simulink model "SPGF_FSK_0000_R2019b"  (R2019b)
settings: Solver=ode3  SolverName=ode4  StartTime=0.0  StopTime=1.4  FixedStep=50e-6/50  RelTol=1e-3  EnableMultiTasking=on
undefined symbols (not defined in the file): D11, Delta
libraries: powerlib x2544, powerlib_meascontrol x204, simulink x24
(part 8 of 33)

== system SPGF_FSK_0000_R2019b/K8/fault ==
  Add : Sum  Inputs=+-
  Arcing : Subsystem  TreatAsAtomicUnit=on
  Constant2 : Constant  Value=FaultPhase
  Control : Product  Inputs=***
  Count Limiter : Subsystem
  Demux : Demux  Outputs=2
  Fault Interruption : Subsystem
  Fault A : Constant  Value=FaultA
  Fault A1 : Constant  Value=0
  Fault A2 : Constant  Value=LimitArcNum
  Fault A3 : Constant  Value=AddTimeDelay
  Fault B : Constant  Value=FaultB
  Fault C : Constant  Value=FaultC
  Ground1 : powerlib/Elements/Ground  LConnTagsString=a
  Ideal Switch A : powerlib/Power Electronics/Ideal Switch  Ron=FaultResistance  Lon=0  IC=0  Rs=SnubberResistance  Cs=SnubberCapacitance  Measurements=on
  Ideal Switch B : powerlib/Power Electronics/Ideal Switch  Ron=FaultResistance  Lon=0  IC=0  Rs=SnubberResistance  Cs=SnubberCapacitance  Measurements=on
  Ideal Switch C : powerlib/Power Electronics/Ideal Switch  Ron=FaultResistance  Lon=0  IC=0  Rs=SnubberResistance  Cs=SnubberCapacitance  Measurements=on
  Mux : Mux  Inputs=2
  Product : Product
  Product1 : Product
  Product2 : Product
  Rground : powerlib/Elements/Series RLC Branch  LConnTagsString=__new0  RConnTagsString=__new0  BranchType=R  Resistance=GroundResistance  Inductance=0  SetiL0=off  InitialCurrent=0  Capacitance=inf  Setx0=off  InitialVoltage=0  Measurements=None
  SW : MultiPortSwitch  DataPortForDefault=Additional data port
  SW_Limit : Switch  Criteria=u2 > Threshold  Threshold=0.5
  SW_TD : Switch  Criteria=u2 > Threshold  Threshold=0.5
  Step : Step  Time=EndFaultTime  SampleTime=0
  Step1 : Step  Time=BeginFaultTime  SampleTime=0
  Time Delay : Subsystem
  A : PMIOPort  Side=Left
  B : PMIOPort  Port=2  Side=Left
  C : PMIOPort  Port=3  Side=Left
  wires:
  Demux/1 -> [I]
  Control/1 -> Time Delay/2(Control), SW_TD/3
  Count Limiter/2(O) -> SW_Limit/1
  Fault A2/1 -> SW_Limit/2
  Arcing/1(O) -> Control/2
  Mux/1 -> Arcing/1(I)
  [V] -> Mux/2
  [I] -> Mux/1
  Add/1 -> Control/1, Arcing/Enable
  Step/1 -> Add/2
  Step1/1 -> Add/1
  Product2/1 -> Ideal Switch C/1
  Fault C/1 -> Product2/2
  Product1/1 -> Ideal Switch B/1
  Fault B/1 -> Product1/2
  Product/1 -> Ideal Switch A/1
  Fault A/1 -> Product/2
  Ideal Switch C/1 -> SW/4
  Ideal Switch B/1 -> SW/3
  Ideal Switch A/1 -> SW/2
  Fault A1/1 -> SW/5
  SW/1 -> Demux/1
  Constant2/1 -> SW/1
  Fault Interruption/1(O) -> Control/3
  SW_Limit/1 -> Product/1, Product1/1, Product2/1
  Fault A3/1 -> SW_TD/2
  SW_TD/1 -> SW_Limit/3, Count Limiter/1(I)
  Count Limiter/1(Count) -> Time Delay/1(Count)
  Time Delay/1(O) -> SW_TD/1
  Demux/2 -> [V]
  connections:
  Ground1/LConn1 -- Rground/RConn1
  Ideal Switch B/RConn1 -- Ideal Switch A/RConn1 -- Rground/LConn1 -- Ideal Switch C/RConn1
  Ideal Switch B/LConn1 -- B/RConn1
  Ideal Switch A/LConn1 -- A/RConn1
  Ideal Switch C/LConn1 -- C/RConn1

== system SPGF_FSK_0000_R2019b/K8/meas ==
  Add : Sum  Inputs=+++
  GainI : Gain
  GainI0 : Gain
  I A: : powerlib/Measurements/Current Measurement  PhasorSimulation=off  OutputType=Complex  PSBequivalent=0
  I B: : powerlib/Measurements/Current Measurement  PhasorSimulation=off  OutputType=Complex  PSBequivalent=0
  I C: : powerlib/Measurements/Current Measurement  PhasorSimulation=off  OutputType=Complex  PSBequivalent=0
  Mux : Mux  Inputs=3
  A : PMIOPort  Side=Left
  B : PMIOPort  Port=2  Side=Left
  C : PMIOPort  Port=3  Side=Left
  a : PMIOPort  Port=4  Side=Right
  b : PMIOPort  Port=5  Side=Right
  c : PMIOPort  Port=6  Side=Right
  tag scope: CT3I0_K8=global, CTIabc_K8=global
  wires:
  I A:/1 -> Mux/1, Add/1
  I B:/1 -> Mux/2, Add/2
  I C:/1 -> Mux/3, Add/3
  Add/1 -> GainI0/1
  GainI0/1 -> [CT3I0_K8]
  Mux/1 -> GainI/1
  GainI/1 -> [CTIabc_K8]
  connections:
  I C:/RConn1 -- c/RConn1
  I B:/RConn1 -- b/RConn1
  a/RConn1 -- I A:/RConn1
  I A:/LConn1 -- A/RConn1
  I C:/LConn1 -- C/RConn1
  I B:/LConn1 -- B/RConn1

== system SPGF_FSK_0000_R2019b/K9/fault ==
  Add : Sum  Inputs=+-
  Arcing : Subsystem  TreatAsAtomicUnit=on
  Constant2 : Constant  Value=FaultPhase
  Control : Product  Inputs=***
  Count Limiter : Subsystem
  Demux : Demux  Outputs=2
  Fault Interruption : Subsystem
  Fault A : Constant  Value=FaultA
  Fault A1 : Constant  Value=0
  Fault A2 : Constant  Value=LimitArcNum
  Fault A3 : Constant  Value=AddTimeDelay
  Fault B : Constant  Value=FaultB
  Fault C : Constant  Value=FaultC
  Ground1 : powerlib/Elements/Ground  LConnTagsString=a
  Ideal Switch A : powerlib/Power Electronics/Ideal Switch  Ron=FaultResistance  Lon=0  IC=0  Rs=SnubberResistance  Cs=SnubberCapacitance  Measurements=on
  Ideal Switch B : powerlib/Power Electronics/Ideal Switch  Ron=FaultResistance  Lon=0  IC=0  Rs=SnubberResistance  Cs=SnubberCapacitance  Measurements=on
  Ideal Switch C : powerlib/Power Electronics/Ideal Switch  Ron=FaultResistance  Lon=0  IC=0  Rs=SnubberResistance  Cs=SnubberCapacitance  Measurements=on
  Mux : Mux  Inputs=2
  Product : Product
  Product1 : Product
  Product2 : Product
  Rground : powerlib/Elements/Series RLC Branch  LConnTagsString=__new0  RConnTagsString=__new0  BranchType=R  Resistance=GroundResistance  Inductance=0  SetiL0=off  InitialCurrent=0  Capacitance=inf  Setx0=off  InitialVoltage=0  Measurements=None
  SW : MultiPortSwitch  DataPortForDefault=Additional data port
  SW_Limit : Switch  Criteria=u2 > Threshold  Threshold=0.5
  SW_TD : Switch  Criteria=u2 > Threshold  Threshold=0.5
  Step : Step  Time=EndFaultTime  SampleTime=0
  Step1 : Step  Time=BeginFaultTime  SampleTime=0
  Time Delay : Subsystem
  A : PMIOPort  Side=Left
  B : PMIOPort  Port=2  Side=Left
  C : PMIOPort  Port=3  Side=Left
  wires:
  Demux/2 -> [V]
  Time Delay/1(O) -> SW_TD/1
  Count Limiter/1(Count) -> Time Delay/1(Count)
  SW_TD/1 -> Count Limiter/1(I), SW_Limit/3
  Fault A3/1 -> SW_TD/2
  SW_Limit/1 -> Product2/1, Product1/1, Product/1
  Fault Interruption/1(O) -> Control/3
  Constant2/1 -> SW/1
  SW/1 -> Demux/1
  Fault A1/1 -> SW/5
  Ideal Switch A/1 -> SW/2
  Ideal Switch B/1 -> SW/3
  Ideal Switch C/1 -> SW/4
  Fault A/1 -> Product/2
  Product/1 -> Ideal Switch A/1
  Fault B/1 -> Product1/2
  Product1/1 -> Ideal Switch B/1
  Fault C/1 -> Product2/2
  Product2/1 -> Ideal Switch C/1
  Step1/1 -> Add/1
  Step/1 -> Add/2
  Add/1 -> Arcing/Enable, Control/1
  [I] -> Mux/1
  [V] -> Mux/2
  Mux/1 -> Arcing/1(I)
  Arcing/1(O) -> Control/2
  Fault A2/1 -> SW_Limit/2
  Count Limiter/2(O) -> SW_Limit/1
  Control/1 -> SW_TD/3, Time Delay/2(Control)
  Demux/1 -> [I]
  connections:
  Ideal Switch C/LConn1 -- C/RConn1
  Ideal Switch A/LConn1 -- A/RConn1
  Ideal Switch B/LConn1 -- B/RConn1
  Ideal Switch C/RConn1 -- Rground/LConn1 -- Ideal Switch A/RConn1 -- Ideal Switch B/RConn1
  Ground1/LConn1 -- Rground/RConn1

== system SPGF_FSK_0000_R2019b/K9/meas ==
  Add : Sum  Inputs=+++
  GainI : Gain
  GainI0 : Gain
  I A: : powerlib/Measurements/Current Measurement  PhasorSimulation=off  OutputType=Complex  PSBequivalent=0
  I B: : powerlib/Measurements/Current Measurement  PhasorSimulation=off  OutputType=Complex  PSBequivalent=0
  I C: : powerlib/Measurements/Current Measurement  PhasorSimulation=off  OutputType=Complex  PSBequivalent=0
  Mux : Mux  Inputs=3
  A : PMIOPort  Side=Left
  B : PMIOPort  Port=2  Side=Left
  C : PMIOPort  Port=3  Side=Left
  a : PMIOPort  Port=4  Side=Right
  b : PMIOPort  Port=5  Side=Right
  c : PMIOPort  Port=6  Side=Right
  tag scope: CT3I0_K9=global, CTIabc_K9=global
  wires:
  GainI/1 -> [CTIabc_K9]
  Mux/1 -> GainI/1
  GainI0/1 -> [CT3I0_K9]
  Add/1 -> GainI0/1
  I C:/1 -> Add/3, Mux/3
  I B:/1 -> Add/2, Mux/2
  I A:/1 -> Add/1, Mux/1
  connections:
  I B:/LConn1 -- B/RConn1
  I C:/LConn1 -- C/RConn1
  I A:/LConn1 -- A/RConn1
  a/RConn1 -- I A:/RConn1
  I B:/RConn1 -- b/RConn1
  I C:/RConn1 -- c/RConn1

== system SPGF_FSK_0000_R2019b/TP11/Nonlinear Load ==
  Cap : powerlib/Elements/Series RLC Branch  LConnTagsString=__new0  RConnTagsString=__new0  BranchType=C  Resistance=34  Inductance=1.04  SetiL0=off  InitialCurrent=0  Capacitance=4e-06  Setx0=off  InitialVoltage=0  Measurements=None
  Cap1 : powerlib/Elements/Series RLC Branch  LConnTagsString=__new0  RConnTagsString=__new0  BranchType=C  Resistance=34  Inductance=1.04  SetiL0=off  InitialCurrent=0  Capacitance=4e-06  Setx0=off  InitialVoltage=0  Measurements=None
  Cap2 : powerlib/Elements/Series RLC Branch  LConnTagsString=__new0  RConnTagsString=__new0  BranchType=C  Resistance=34  Inductance=1.04  SetiL0=off  InitialCurrent=0  Capacitance=4e-06  Setx0=off  InitialVoltage=0  Measurements=None
  Ground : powerlib/Elements/Ground  LConnTagsString=a
  RL : powerlib/Elements/Series RLC Branch  LConnTagsString=__new0  RConnTagsString=__new0  BranchType=RL  Resistance=58  Inductance=1.04  SetiL0=off  InitialCurrent=0  Capacitance=1e-6  Setx0=off  InitialVoltage=0  Measurements=None
  RL1 : powerlib/Elements/Series RLC Branch  LConnTagsString=__new0  RConnTagsString=__new0  BranchType=RL  Resistance=40  Inductance=1.04  SetiL0=off  InitialCurrent=0  Capacitance=1e-6  Setx0=off  InitialVoltage=0  Measurements=None
  RL2 : powerlib/Elements/Series RLC Branch  LConnTagsString=__new0  RConnTagsString=__new0  BranchType=RL  Resistance=40  Inductance=1.04  SetiL0=off  InitialCurrent=0  Capacitance=1e-6  Setx0=off  InitialVoltage=0  Measurements=None
  Universal Bridge : powerlib/Power Electronics/Universal Bridge  Arms=2  SnubberResistance=1e5  SnubberCapacitance=inf  Device=Diodes  Ron=1e-3  Lon=0  ForwardVoltages="[  0  0  ]"  ForwardVoltage=-160  GTOparameters=[ 10e-6 , 20e-6 ]  IGBTparameters=[ 1e-6 , 2e-6 ]  Measurements=None  Measurements_2=None  converterType=Rectifier
  Universal Bridge1 : powerlib/Power Electronics/Universal Bridge  Arms=2  SnubberResistance=1e5  SnubberCapacitance=inf  Device=Diodes  Ron=1e-3  Lon=0  ForwardVoltages="[  0  0  ]"  ForwardVoltage=-160  GTOparameters=[ 10e-6 , 20e-6 ]  IGBTparameters=[ 1e-6 , 2e-6 ]  Measurements=None  Measurements_2=None  converterType=Rectifier
  Universal Bridge2 : powerlib/Power Electronics/Universal Bridge  Arms=2  SnubberResistance=1e5  SnubberCapacitance=inf  Device=Diodes  Ron=1e-3  Lon=0  ForwardVoltages="[  0  0  ]"  ForwardVoltage=-160  GTOparameters=[ 10e-6 , 20e-6 ]  IGBTparameters=[ 1e-6 , 2e-6 ]  Measurements=None  Measurements_2=None  converterType=Rectifier
  A : PMIOPort  Side=Left
  B : PMIOPort  Port=2  Side=Left
  C : PMIOPort  Port=3  Side=Left
  connections:
  Cap/LConn1 -- Universal Bridge/RConn1 -- RL/LConn1
  Cap/RConn1 -- RL/RConn1 -- Universal Bridge/RConn2
  Cap1/LConn1 -- Universal Bridge1/RConn1 -- RL1/LConn1
  Universal Bridge1/RConn2 -- RL1/RConn1 -- Cap1/RConn1
  Cap2/LConn1 -- Universal Bridge2/RConn1 -- RL2/LConn1
  Cap2/RConn1 -- Universal Bridge2/RConn2 -- RL2/RConn1
  Universal Bridge/LConn1 -- A/RConn1
  Universal Bridge1/LConn1 -- B/RConn1
  Universal Bridge2/LConn1 -- C/RConn1
  Ground/LConn1 -- Universal Bridge/LConn2 -- Universal Bridge1/LConn2 -- Universal Bridge2/LConn2

== system SPGF_FSK_0000_R2019b/TP11/Nonlinear Load 3ph ==
  Cap : powerlib/Elements/Series RLC Branch  LConnTagsString=__new0  RConnTagsString=__new0  BranchType=C  Resistance=34  Inductance=1.04  SetiL0=off  InitialCurrent=0  Capacitance=4e-06  Setx0=off  InitialVoltage=0  Measurements=None
  RL : powerlib/Elements/Series RLC Branch  LConnTagsString=__new0  RConnTagsString=__new0  BranchType=RL  Resistance=58  Inductance=1.04  SetiL0=off  InitialCurrent=0  Capacitance=1e-6  Setx0=off  InitialVoltage=0  Measurements=None
  Universal Bridge : powerlib/Power Electronics/Universal Bridge  Arms=3  SnubberResistance=1e5  SnubberCapacitance=inf  Device=Diodes  Ron=1e-3  Lon=0  ForwardVoltages="[  0  0  ]"  ForwardVoltage=-160  GTOparameters=[ 10e-6 , 20e-6 ]  IGBTparameters=[ 1e-6 , 2e-6 ]  Measurements=None  Measurements_2=None  converterType=Rectifier
  A : PMIOPort  Side=Left
  B : PMIOPort  Port=2  Side=Left
  C : PMIOPort  Port=3  Side=Left
  connections:
  Universal Bridge/RConn1 -- RL/LConn1 -- Cap/LConn1
  Cap/RConn1 -- Universal Bridge/RConn2 -- RL/RConn1
  Universal Bridge/LConn2 -- B/RConn1
  C/RConn1 -- Universal Bridge/LConn3
  A/RConn1 -- Universal Bridge/LConn1

== system SPGF_FSK_0000_R2019b/TP11/Q ==
  breaker : Subsystem  Commented=on  mask{SwitchA=off, SwitchB=off, SwitchC=off, InitialStatus=[1 1 1], BreakerResistance=0.0001, SnubberResistance=1e6, SnubberCapacitance=inf, TransitionTimes=[0.5 0.7], ShiftTimes=[0 0 0]}
      mask prompts: SwitchA "Switching of phase A"; SwitchB "Switching of phase B"; SwitchC "Switching of phase C"; InitialStatus "Initial status of phase breaker [A, B, C]"; BreakerResistance "Breaker resistance Ron (ohms) :"; SnubberResistance "Snubbers resistance Rp (ohms) :"; SnubberCapacitance "Snubbers capacitance Cp (F) :"; TransitionTimes "Transition times (s) :"; ShiftTimes "Time differences for switch [tA, tB, tC] (s) :"
      mask init: same as SPGF_FSK_0000_R2019b/Feed/Q/breaker
      mask Display:
      | % port_label('input',1,'Iabc');
      | 
      | port_label('lconn',1,'A');
      | port_label('lconn',2,'B');
      | port_label('lconn',3,'C');
      | 
      | port_label('rconn',1,'a');
      | port_label('rconn',2,'b');
      | port_label('rconn',3,'c');
      | 
      | disp('   Q    ');
  meas : Subsystem
  shunt : Subsystem
  A : PMIOPort  Side=Right
  B : PMIOPort  Port=2  Side=Right
  C : PMIOPort  Port=3  Side=Right
  a : PMIOPort  Port=4  Side=Left
  b : PMIOPort  Port=5  Side=Left
  c : PMIOPort  Port=6  Side=Left
  connections:
  shunt/LConn3 -- C/RConn1 -- breaker/LConn3
  shunt/LConn2 -- B/RConn1 -- breaker/LConn2
  A/RConn1 -- shunt/LConn1 -- breaker/LConn1
  meas/RConn1 -- a/RConn1
  meas/RConn2 -- b/RConn1
  meas/RConn3 -- c/RConn1
  meas/LConn3 -- breaker/RConn3 -- shunt/RConn3
  meas/LConn2 -- breaker/RConn2 -- shunt/RConn2
  meas/LConn1 -- breaker/RConn1 -- shunt/RConn1

== system SPGF_FSK_0000_R2019b/TP12/Nonlinear Load ==
  Cap : powerlib/Elements/Series RLC Branch  LConnTagsString=__new0  RConnTagsString=__new0  BranchType=C  Resistance=34  Inductance=1.04  SetiL0=off  InitialCurrent=0  Capacitance=4e-06  Setx0=off  InitialVoltage=0  Measurements=None
  Cap1 : powerlib/Elements/Series RLC Branch  LConnTagsString=__new0  RConnTagsString=__new0  BranchType=C  Resistance=34  Inductance=1.04  SetiL0=off  InitialCurrent=0  Capacitance=4e-06  Setx0=off  InitialVoltage=0  Measurements=None
  Cap2 : powerlib/Elements/Series RLC Branch  LConnTagsString=__new0  RConnTagsString=__new0  BranchType=C  Resistance=34  Inductance=1.04  SetiL0=off  InitialCurrent=0  Capacitance=4e-06  Setx0=off  InitialVoltage=0  Measurements=None
  Ground : powerlib/Elements/Ground  LConnTagsString=a
  RL : powerlib/Elements/Series RLC Branch  LConnTagsString=__new0  RConnTagsString=__new0  BranchType=RL  Resistance=58  Inductance=1.04  SetiL0=off  InitialCurrent=0  Capacitance=1e-6  Setx0=off  InitialVoltage=0  Measurements=None
  RL1 : powerlib/Elements/Series RLC Branch  LConnTagsString=__new0  RConnTagsString=__new0  BranchType=RL  Resistance=40  Inductance=1.04  SetiL0=off  InitialCurrent=0  Capacitance=1e-6  Setx0=off  InitialVoltage=0  Measurements=None
  RL2 : powerlib/Elements/Series RLC Branch  LConnTagsString=__new0  RConnTagsString=__new0  BranchType=RL  Resistance=40  Inductance=1.04  SetiL0=off  InitialCurrent=0  Capacitance=1e-6  Setx0=off  InitialVoltage=0  Measurements=None
  Universal Bridge : powerlib/Power Electronics/Universal Bridge  Arms=2  SnubberResistance=1e5  SnubberCapacitance=inf  Device=Diodes  Ron=1e-3  Lon=0  ForwardVoltages="[  0  0  ]"  ForwardVoltage=-160  GTOparameters=[ 10e-6 , 20e-6 ]  IGBTparameters=[ 1e-6 , 2e-6 ]  Measurements=None  Measurements_2=None  converterType=Rectifier
  Universal Bridge1 : powerlib/Power Electronics/Universal Bridge  Arms=2  SnubberResistance=1e5  SnubberCapacitance=inf  Device=Diodes  Ron=1e-3  Lon=0  ForwardVoltages="[  0  0  ]"  ForwardVoltage=-160  GTOparameters=[ 10e-6 , 20e-6 ]  IGBTparameters=[ 1e-6 , 2e-6 ]  Measurements=None  Measurements_2=None  converterType=Rectifier
  Universal Bridge2 : powerlib/Power Electronics/Universal Bridge  Arms=2  SnubberResistance=1e5  SnubberCapacitance=inf  Device=Diodes  Ron=1e-3  Lon=0  ForwardVoltages="[  0  0  ]"  ForwardVoltage=-160  GTOparameters=[ 10e-6 , 20e-6 ]  IGBTparameters=[ 1e-6 , 2e-6 ]  Measurements=None  Measurements_2=None  converterType=Rectifier
  A : PMIOPort  Side=Left
  B : PMIOPort  Port=2  Side=Left
  C : PMIOPort  Port=3  Side=Left
  connections:
  Cap/LConn1 -- Universal Bridge/RConn1 -- RL/LConn1
  Cap/RConn1 -- RL/RConn1 -- Universal Bridge/RConn2
  Cap1/LConn1 -- Universal Bridge1/RConn1 -- RL1/LConn1
  Universal Bridge1/RConn2 -- RL1/RConn1 -- Cap1/RConn1
  Cap2/LConn1 -- Universal Bridge2/RConn1 -- RL2/LConn1
  Cap2/RConn1 -- Universal Bridge2/RConn2 -- RL2/RConn1
  Universal Bridge/LConn1 -- A/RConn1
  Universal Bridge1/LConn1 -- B/RConn1
  Universal Bridge2/LConn1 -- C/RConn1
  Ground/LConn1 -- Universal Bridge/LConn2 -- Universal Bridge1/LConn2 -- Universal Bridge2/LConn2

== system SPGF_FSK_0000_R2019b/TP12/Nonlinear Load 3ph ==
  Cap : powerlib/Elements/Series RLC Branch  LConnTagsString=__new0  RConnTagsString=__new0  BranchType=C  Resistance=34  Inductance=1.04  SetiL0=off  InitialCurrent=0  Capacitance=4e-06  Setx0=off  InitialVoltage=0  Measurements=None
  RL : powerlib/Elements/Series RLC Branch  LConnTagsString=__new0  RConnTagsString=__new0  BranchType=RL  Resistance=58  Inductance=1.04  SetiL0=off  InitialCurrent=0  Capacitance=1e-6  Setx0=off  InitialVoltage=0  Measurements=None
  Universal Bridge : powerlib/Power Electronics/Universal Bridge  Arms=3  SnubberResistance=1e5  SnubberCapacitance=inf  Device=Diodes  Ron=1e-3  Lon=0  ForwardVoltages="[  0  0  ]"  ForwardVoltage=-160  GTOparameters=[ 10e-6 , 20e-6 ]  IGBTparameters=[ 1e-6 , 2e-6 ]  Measurements=None  Measurements_2=None  converterType=Rectifier
  A : PMIOPort  Side=Left
  B : PMIOPort  Port=2  Side=Left
  C : PMIOPort  Port=3  Side=Left
  connections:
  Universal Bridge/RConn1 -- RL/LConn1 -- Cap/LConn1
  Cap/RConn1 -- Universal Bridge/RConn2 -- RL/RConn1
  Universal Bridge/LConn2 -- B/RConn1
  C/RConn1 -- Universal Bridge/LConn3
  A/RConn1 -- Universal Bridge/LConn1

== system SPGF_FSK_0000_R2019b/TP12/Q ==
  breaker : Subsystem  Commented=on  mask{SwitchA=off, SwitchB=off, SwitchC=off, InitialStatus=[1 1 1], BreakerResistance=0.0001, SnubberResistance=1e6, SnubberCapacitance=inf, TransitionTimes=[0.5 0.7], ShiftTimes=[0 0 0]}
      mask prompts: SwitchA "Switching of phase A"; SwitchB "Switching of phase B"; SwitchC "Switching of phase C"; InitialStatus "Initial status of phase breaker [A, B, C]"; BreakerResistance "Breaker resistance Ron (ohms) :"; SnubberResistance "Snubbers resistance Rp (ohms) :"; SnubberCapacitance "Snubbers capacitance Cp (F) :"; TransitionTimes "Transition times (s) :"; ShiftTimes "Time differences for switch [tA, tB, tC] (s) :"
      mask init: same as SPGF_FSK_0000_R2019b/Feed/Q/breaker
      mask Display:
      | % port_label('input',1,'Iabc');
      | 
      | port_label('lconn',1,'A');
      | port_label('lconn',2,'B');
      | port_label('lconn',3,'C');
      | 
      | port_label('rconn',1,'a');
      | port_label('rconn',2,'b');
      | port_label('rconn',3,'c');
      | 
      | disp('   Q    ');
  meas : Subsystem
  shunt : Subsystem
  A : PMIOPort  Side=Right
  B : PMIOPort  Port=2  Side=Right
  C : PMIOPort  Port=3  Side=Right
  a : PMIOPort  Port=4  Side=Left
  b : PMIOPort  Port=5  Side=Left
  c : PMIOPort  Port=6  Side=Left
  connections:
  shunt/LConn3 -- C/RConn1 -- breaker/LConn3
  shunt/LConn2 -- B/RConn1 -- breaker/LConn2
  A/RConn1 -- shunt/LConn1 -- breaker/LConn1
  meas/RConn1 -- a/RConn1
  meas/RConn2 -- b/RConn1
  meas/RConn3 -- c/RConn1
  meas/LConn3 -- breaker/RConn3 -- shunt/RConn3
  meas/LConn2 -- breaker/RConn2 -- shunt/RConn2
  meas/LConn1 -- breaker/RConn1 -- shunt/RConn1

== system SPGF_FSK_0000_R2019b/TP13/Nonlinear Load ==
  Cap : powerlib/Elements/Series RLC Branch  LConnTagsString=__new0  RConnTagsString=__new0  BranchType=C  Resistance=34  Inductance=1.04  SetiL0=off  InitialCurrent=0  Capacitance=4e-06  Setx0=off  InitialVoltage=0  Measurements=None
  Cap1 : powerlib/Elements/Series RLC Branch  LConnTagsString=__new0  RConnTagsString=__new0  BranchType=C  Resistance=34  Inductance=1.04  SetiL0=off  InitialCurrent=0  Capacitance=4e-06  Setx0=off  InitialVoltage=0  Measurements=None
  Cap2 : powerlib/Elements/Series RLC Branch  LConnTagsString=__new0  RConnTagsString=__new0  BranchType=C  Resistance=34  Inductance=1.04  SetiL0=off  InitialCurrent=0  Capacitance=4e-06  Setx0=off  InitialVoltage=0  Measurements=None
  Ground : powerlib/Elements/Ground  LConnTagsString=a
  RL : powerlib/Elements/Series RLC Branch  LConnTagsString=__new0  RConnTagsString=__new0  BranchType=RL  Resistance=58  Inductance=1.04  SetiL0=off  InitialCurrent=0  Capacitance=1e-6  Setx0=off  InitialVoltage=0  Measurements=None
  RL1 : powerlib/Elements/Series RLC Branch  LConnTagsString=__new0  RConnTagsString=__new0  BranchType=RL  Resistance=40  Inductance=1.04  SetiL0=off  InitialCurrent=0  Capacitance=1e-6  Setx0=off  InitialVoltage=0  Measurements=None
  RL2 : powerlib/Elements/Series RLC Branch  LConnTagsString=__new0  RConnTagsString=__new0  BranchType=RL  Resistance=40  Inductance=1.04  SetiL0=off  InitialCurrent=0  Capacitance=1e-6  Setx0=off  InitialVoltage=0  Measurements=None
  Universal Bridge : powerlib/Power Electronics/Universal Bridge  Arms=2  SnubberResistance=1e5  SnubberCapacitance=inf  Device=Diodes  Ron=1e-3  Lon=0  ForwardVoltages="[  0  0  ]"  ForwardVoltage=-160  GTOparameters=[ 10e-6 , 20e-6 ]  IGBTparameters=[ 1e-6 , 2e-6 ]  Measurements=None  Measurements_2=None  converterType=Rectifier
  Universal Bridge1 : powerlib/Power Electronics/Universal Bridge  Arms=2  SnubberResistance=1e5  SnubberCapacitance=inf  Device=Diodes  Ron=1e-3  Lon=0  ForwardVoltages="[  0  0  ]"  ForwardVoltage=-160  GTOparameters=[ 10e-6 , 20e-6 ]  IGBTparameters=[ 1e-6 , 2e-6 ]  Measurements=None  Measurements_2=None  converterType=Rectifier
  Universal Bridge2 : powerlib/Power Electronics/Universal Bridge  Arms=2  SnubberResistance=1e5  SnubberCapacitance=inf  Device=Diodes  Ron=1e-3  Lon=0  ForwardVoltages="[  0  0  ]"  ForwardVoltage=-160  GTOparameters=[ 10e-6 , 20e-6 ]  IGBTparameters=[ 1e-6 , 2e-6 ]  Measurements=None  Measurements_2=None  converterType=Rectifier
  A : PMIOPort  Side=Left
  B : PMIOPort  Port=2  Side=Left
  C : PMIOPort  Port=3  Side=Left
  connections:
  Cap/LConn1 -- Universal Bridge/RConn1 -- RL/LConn1
  Cap/RConn1 -- RL/RConn1 -- Universal Bridge/RConn2
  Cap1/LConn1 -- Universal Bridge1/RConn1 -- RL1/LConn1
  Universal Bridge1/RConn2 -- RL1/RConn1 -- Cap1/RConn1
  Cap2/LConn1 -- Universal Bridge2/RConn1 -- RL2/LConn1
  Cap2/RConn1 -- Universal Bridge2/RConn2 -- RL2/RConn1
  Universal Bridge/LConn1 -- A/RConn1
  Universal Bridge1/LConn1 -- B/RConn1
  Universal Bridge2/LConn1 -- C/RConn1
  Ground/LConn1 -- Universal Bridge/LConn2 -- Universal Bridge1/LConn2 -- Universal Bridge2/LConn2

== system SPGF_FSK_0000_R2019b/TP13/Nonlinear Load 3ph ==
  Cap : powerlib/Elements/Series RLC Branch  LConnTagsString=__new0  RConnTagsString=__new0  BranchType=C  Resistance=34  Inductance=1.04  SetiL0=off  InitialCurrent=0  Capacitance=4e-06  Setx0=off  InitialVoltage=0  Measurements=None
  RL : powerlib/Elements/Series RLC Branch  LConnTagsString=__new0  RConnTagsString=__new0  BranchType=RL  Resistance=58  Inductance=1.04  SetiL0=off  InitialCurrent=0  Capacitance=1e-6  Setx0=off  InitialVoltage=0  Measurements=None
  Universal Bridge : powerlib/Power Electronics/Universal Bridge  Arms=3  SnubberResistance=1e5  SnubberCapacitance=inf  Device=Diodes  Ron=1e-3  Lon=0  ForwardVoltages="[  0  0  ]"  ForwardVoltage=-160  GTOparameters=[ 10e-6 , 20e-6 ]  IGBTparameters=[ 1e-6 , 2e-6 ]  Measurements=None  Measurements_2=None  converterType=Rectifier
  A : PMIOPort  Side=Left
  B : PMIOPort  Port=2  Side=Left
  C : PMIOPort  Port=3  Side=Left
  connections:
  Universal Bridge/RConn1 -- RL/LConn1 -- Cap/LConn1
  Cap/RConn1 -- Universal Bridge/RConn2 -- RL/RConn1
  Universal Bridge/LConn2 -- B/RConn1
  C/RConn1 -- Universal Bridge/LConn3
  A/RConn1 -- Universal Bridge/LConn1

== system SPGF_FSK_0000_R2019b/TP13/Q ==
  breaker : Subsystem  Commented=on  mask{SwitchA=off, SwitchB=off, SwitchC=off, InitialStatus=[1 1 1], BreakerResistance=0.0001, SnubberResistance=1e6, SnubberCapacitance=inf, TransitionTimes=[0.5 0.7], ShiftTimes=[0 0 0]}
      mask prompts: SwitchA "Switching of phase A"; SwitchB "Switching of phase B"; SwitchC "Switching of phase C"; InitialStatus "Initial status of phase breaker [A, B, C]"; BreakerResistance "Breaker resistance Ron (ohms) :"; SnubberResistance "Snubbers resistance Rp (ohms) :"; SnubberCapacitance "Snubbers capacitance Cp (F) :"; TransitionTimes "Transition times (s) :"; ShiftTimes "Time differences for switch [tA, tB, tC] (s) :"
      mask init: same as SPGF_FSK_0000_R2019b/Feed/Q/breaker
      mask Display:
      | % port_label('input',1,'Iabc');
      | 
      | port_label('lconn',1,'A');
      | port_label('lconn',2,'B');
      | port_label('lconn',3,'C');
      | 
      | port_label('rconn',1,'a');
      | port_label('rconn',2,'b');
      | port_label('rconn',3,'c');
      | 
      | disp('   Q    ');
  meas : Subsystem
  shunt : Subsystem
  A : PMIOPort  Side=Right
  B : PMIOPort  Port=2  Side=Right
  C : PMIOPort  Port=3  Side=Right
  a : PMIOPort  Port=4  Side=Left
  b : PMIOPort  Port=5  Side=Left
  c : PMIOPort  Port=6  Side=Left
  connections:
  shunt/LConn3 -- C/RConn1 -- breaker/LConn3
  shunt/LConn2 -- B/RConn1 -- breaker/LConn2
  A/RConn1 -- shunt/LConn1 -- breaker/LConn1
  meas/RConn1 -- a/RConn1
  meas/RConn2 -- b/RConn1
  meas/RConn3 -- c/RConn1
  meas/LConn3 -- breaker/RConn3 -- shunt/RConn3
  meas/LConn2 -- breaker/RConn2 -- shunt/RConn2
  meas/LConn1 -- breaker/RConn1 -- shunt/RConn1

== system SPGF_FSK_0000_R2019b/TP14/Nonlinear Load ==
  Cap : powerlib/Elements/Series RLC Branch  LConnTagsString=__new0  RConnTagsString=__new0  BranchType=C  Resistance=34  Inductance=1.04  SetiL0=off  InitialCurrent=0  Capacitance=4e-06  Setx0=off  InitialVoltage=0  Measurements=None
  Cap1 : powerlib/Elements/Series RLC Branch  LConnTagsString=__new0  RConnTagsString=__new0  BranchType=C  Resistance=34  Inductance=1.04  SetiL0=off  InitialCurrent=0  Capacitance=4e-06  Setx0=off  InitialVoltage=0  Measurements=None
  Cap2 : powerlib/Elements/Series RLC Branch  LConnTagsString=__new0  RConnTagsString=__new0  BranchType=C  Resistance=34  Inductance=1.04  SetiL0=off  InitialCurrent=0  Capacitance=4e-06  Setx0=off  InitialVoltage=0  Measurements=None
  Ground : powerlib/Elements/Ground  LConnTagsString=a
  RL : powerlib/Elements/Series RLC Branch  LConnTagsString=__new0  RConnTagsString=__new0  BranchType=RL  Resistance=58  Inductance=1.04  SetiL0=off  InitialCurrent=0  Capacitance=1e-6  Setx0=off  InitialVoltage=0  Measurements=None
  RL1 : powerlib/Elements/Series RLC Branch  LConnTagsString=__new0  RConnTagsString=__new0  BranchType=RL  Resistance=40  Inductance=1.04  SetiL0=off  InitialCurrent=0  Capacitance=1e-6  Setx0=off  InitialVoltage=0  Measurements=None
  RL2 : powerlib/Elements/Series RLC Branch  LConnTagsString=__new0  RConnTagsString=__new0  BranchType=RL  Resistance=40  Inductance=1.04  SetiL0=off  InitialCurrent=0  Capacitance=1e-6  Setx0=off  InitialVoltage=0  Measurements=None
  Universal Bridge : powerlib/Power Electronics/Universal Bridge  Arms=2  SnubberResistance=1e5  SnubberCapacitance=inf  Device=Diodes  Ron=1e-3  Lon=0  ForwardVoltages="[  0  0  ]"  ForwardVoltage=-160  GTOparameters=[ 10e-6 , 20e-6 ]  IGBTparameters=[ 1e-6 , 2e-6 ]  Measurements=None  Measurements_2=None  converterType=Rectifier
  Universal Bridge1 : powerlib/Power Electronics/Universal Bridge  Arms=2  SnubberResistance=1e5  SnubberCapacitance=inf  Device=Diodes  Ron=1e-3  Lon=0  ForwardVoltages="[  0  0  ]"  ForwardVoltage=-160  GTOparameters=[ 10e-6 , 20e-6 ]  IGBTparameters=[ 1e-6 , 2e-6 ]  Measurements=None  Measurements_2=None  converterType=Rectifier
  Universal Bridge2 : powerlib/Power Electronics/Universal Bridge  Arms=2  SnubberResistance=1e5  SnubberCapacitance=inf  Device=Diodes  Ron=1e-3  Lon=0  ForwardVoltages="[  0  0  ]"  ForwardVoltage=-160  GTOparameters=[ 10e-6 , 20e-6 ]  IGBTparameters=[ 1e-6 , 2e-6 ]  Measurements=None  Measurements_2=None  converterType=Rectifier
  A : PMIOPort  Side=Left
  B : PMIOPort  Port=2  Side=Left
  C : PMIOPort  Port=3  Side=Left
  connections:
  Cap/LConn1 -- Universal Bridge/RConn1 -- RL/LConn1
  Cap/RConn1 -- RL/RConn1 -- Universal Bridge/RConn2
  Cap1/LConn1 -- Universal Bridge1/RConn1 -- RL1/LConn1
  Universal Bridge1/RConn2 -- RL1/RConn1 -- Cap1/RConn1
  Cap2/LConn1 -- Universal Bridge2/RConn1 -- RL2/LConn1
  Cap2/RConn1 -- Universal Bridge2/RConn2 -- RL2/RConn1
  Universal Bridge/LConn1 -- A/RConn1
  Universal Bridge1/LConn1 -- B/RConn1
  Universal Bridge2/LConn1 -- C/RConn1
  Ground/LConn1 -- Universal Bridge/LConn2 -- Universal Bridge1/LConn2 -- Universal Bridge2/LConn2

== system SPGF_FSK_0000_R2019b/TP14/Nonlinear Load 3ph ==
  Cap : powerlib/Elements/Series RLC Branch  LConnTagsString=__new0  RConnTagsString=__new0  BranchType=C  Resistance=34  Inductance=1.04  SetiL0=off  InitialCurrent=0  Capacitance=4e-06  Setx0=off  InitialVoltage=0  Measurements=None
  RL : powerlib/Elements/Series RLC Branch  LConnTagsString=__new0  RConnTagsString=__new0  BranchType=RL  Resistance=58  Inductance=1.04  SetiL0=off  InitialCurrent=0  Capacitance=1e-6  Setx0=off  InitialVoltage=0  Measurements=None
  Universal Bridge : powerlib/Power Electronics/Universal Bridge  Arms=3  SnubberResistance=1e5  SnubberCapacitance=inf  Device=Diodes  Ron=1e-3  Lon=0  ForwardVoltages="[  0  0  ]"  ForwardVoltage=-160  GTOparameters=[ 10e-6 , 20e-6 ]  IGBTparameters=[ 1e-6 , 2e-6 ]  Measurements=None  Measurements_2=None  converterType=Rectifier
  A : PMIOPort  Side=Left
  B : PMIOPort  Port=2  Side=Left
  C : PMIOPort  Port=3  Side=Left
  connections:
  Universal Bridge/RConn1 -- RL/LConn1 -- Cap/LConn1
  Cap/RConn1 -- Universal Bridge/RConn2 -- RL/RConn1
  Universal Bridge/LConn2 -- B/RConn1
  C/RConn1 -- Universal Bridge/LConn3
  A/RConn1 -- Universal Bridge/LConn1

== system SPGF_FSK_0000_R2019b/TP14/Q ==
  breaker : Subsystem  Commented=on  mask{SwitchA=off, SwitchB=off, SwitchC=off, InitialStatus=[1 1 1], BreakerResistance=0.0001, SnubberResistance=1e6, SnubberCapacitance=inf, TransitionTimes=[0.5 0.7], ShiftTimes=[0 0 0]}
      mask prompts: SwitchA "Switching of phase A"; SwitchB "Switching of phase B"; SwitchC "Switching of phase C"; InitialStatus "Initial status of phase breaker [A, B, C]"; BreakerResistance "Breaker resistance Ron (ohms) :"; SnubberResistance "Snubbers resistance Rp (ohms) :"; SnubberCapacitance "Snubbers capacitance Cp (F) :"; TransitionTimes "Transition times (s) :"; ShiftTimes "Time differences for switch [tA, tB, tC] (s) :"
      mask init: same as SPGF_FSK_0000_R2019b/Feed/Q/breaker
      mask Display:
      | % port_label('input',1,'Iabc');
      | 
      | port_label('lconn',1,'A');
      | port_label('lconn',2,'B');
      | port_label('lconn',3,'C');
      | 
      | port_label('rconn',1,'a');
      | port_label('rconn',2,'b');
      | port_label('rconn',3,'c');
      | 
      | disp('   Q    ');
  meas : Subsystem
  shunt : Subsystem
  A : PMIOPort  Side=Right
  B : PMIOPort  Port=2  Side=Right
  C : PMIOPort  Port=3  Side=Right
  a : PMIOPort  Port=4  Side=Left
  b : PMIOPort  Port=5  Side=Left
  c : PMIOPort  Port=6  Side=Left
  connections:
  shunt/LConn3 -- C/RConn1 -- breaker/LConn3
  shunt/LConn2 -- B/RConn1 -- breaker/LConn2
  A/RConn1 -- shunt/LConn1 -- breaker/LConn1
  meas/RConn1 -- a/RConn1
  meas/RConn2 -- b/RConn1
  meas/RConn3 -- c/RConn1
  meas/LConn3 -- breaker/RConn3 -- shunt/RConn3
  meas/LConn2 -- breaker/RConn2 -- shunt/RConn2
  meas/LConn1 -- breaker/RConn1 -- shunt/RConn1

== system SPGF_FSK_0000_R2019b/TP15/Fourier Block ==
  abc : Inport
  Scope{2..11} (10 alike) : Scope
  Sequence Analyzer : powerlib_meascontrol/Measurements/Sequence Analyzer  Freq=50  n=1  seq=Positive  InInit=[0, 0]  Ts=0
  Sequence Analyzer1 : powerlib_meascontrol/Measurements/Sequence Analyzer  Freq=50  n=2  seq=Positive  InInit=[0, 0]  Ts=0
  Sequence Analyzer2 : powerlib_meascontrol/Measurements/Sequence Analyzer  Freq=50  n=3  seq=Positive  InInit=[0, 0]  Ts=0
  Sequence Analyzer3 : powerlib_meascontrol/Measurements/Sequence Analyzer  Freq=50  n=5  seq=Positive  InInit=[0, 0]  Ts=0
  Sequence Analyzer4 : powerlib_meascontrol/Measurements/Sequence Analyzer  Freq=50  n=7  seq=Positive  InInit=[0, 0]  Ts=0
  Sequence Analyzer5 : powerlib_meascontrol/Measurements/Sequence Analyzer  Freq=50  n=9  seq=Positive  InInit=[0, 0]  Ts=0
  Sequence Analyzer6 : powerlib_meascontrol/Measurements/Sequence Analyzer  Freq=50  n=11  seq=Positive  InInit=[0, 0]  Ts=0
  Sequence Analyzer7 : powerlib_meascontrol/Measurements/Sequence Analyzer  Freq=50  n=13  seq=Positive  InInit=[0, 0]  Ts=0
  Sequence Analyzer8 : powerlib_meascontrol/Measurements/Sequence Analyzer  Freq=50  n=15  seq=Positive  InInit=[0, 0]  Ts=0
  Sequence Analyzer9 : powerlib_meascontrol/Measurements/Sequence Analyzer  Freq=50  n=17  seq=Positive  InInit=[0, 0]  Ts=0
  Terminator{,1..9} (10 alike) : Terminator
  wires:
  Sequence Analyzer4/1 -> Scope6/1
  Sequence Analyzer3/1 -> Scope5/1
  Sequence Analyzer5/1 -> Scope7/1
  abc/1 -> Sequence Analyzer9/1, Sequence Analyzer8/1, Sequence Analyzer7/1, Sequence Analyzer6/1, Sequence Analyzer5/1, Sequence Analyzer4/1, Sequence Analyzer2/1, Sequence Analyzer1/1, Sequence Analyzer/1, Sequence Analyzer3/1
  Sequence Analyzer1/1 -> Scope3/1
  Sequence Analyzer9/2 -> Terminator9/1
  Sequence Analyzer2/1 -> Scope4/1
  Sequence Analyzer/1 -> Scope2/1
  Sequence Analyzer3/2 -> Terminator5/1
  Sequence Analyzer4/2 -> Terminator4/1
  Sequence Analyzer5/2 -> Terminator3/1
  Sequence Analyzer1/2 -> Terminator1/1
  Sequence Analyzer/2 -> Terminator2/1
  Sequence Analyzer8/2 -> Terminator6/1
  Sequence Analyzer6/2 -> Terminator8/1
  Sequence Analyzer7/2 -> Terminator7/1
  Sequence Analyzer2/2 -> Terminator/1
  Sequence Analyzer9/1 -> Scope11/1
  Sequence Analyzer6/1 -> Scope8/1
  Sequence Analyzer8/1 -> Scope10/1
  Sequence Analyzer7/1 -> Scope9/1

== system SPGF_FSK_0000_R2019b/TP15/Fourier Block1 ==
  abc : Inport
  Scope{2..11} (10 alike) : Scope
  Sequence Analyzer : powerlib_meascontrol/Measurements/Sequence Analyzer  Freq=50  n=1  seq=Positive  InInit=[0, 0]  Ts=0
  Sequence Analyzer1 : powerlib_meascontrol/Measurements/Sequence Analyzer  Freq=50  n=2  seq=Positive  InInit=[0, 0]  Ts=0
  Sequence Analyzer2 : powerlib_meascontrol/Measurements/Sequence Analyzer  Freq=50  n=3  seq=Positive  InInit=[0, 0]  Ts=0
  Sequence Analyzer3 : powerlib_meascontrol/Measurements/Sequence Analyzer  Freq=50  n=5  seq=Positive  InInit=[0, 0]  Ts=0
  Sequence Analyzer4 : powerlib_meascontrol/Measurements/Sequence Analyzer  Freq=50  n=7  seq=Positive  InInit=[0, 0]  Ts=0
  Sequence Analyzer5 : powerlib_meascontrol/Measurements/Sequence Analyzer  Freq=50  n=9  seq=Positive  InInit=[0, 0]  Ts=0
  Sequence Analyzer6 : powerlib_meascontrol/Measurements/Sequence Analyzer  Freq=50  n=11  seq=Positive  InInit=[0, 0]  Ts=0
  Sequence Analyzer7 : powerlib_meascontrol/Measurements/Sequence Analyzer  Freq=50  n=13  seq=Positive  InInit=[0, 0]  Ts=0
  Sequence Analyzer8 : powerlib_meascontrol/Measurements/Sequence Analyzer  Freq=50  n=15  seq=Positive  InInit=[0, 0]  Ts=0
  Sequence Analyzer9 : powerlib_meascontrol/Measurements/Sequence Analyzer  Freq=50  n=17  seq=Positive  InInit=[0, 0]  Ts=0
  Terminator{,1..9} (10 alike) : Terminator
  wires:
  Sequence Analyzer7/1 -> Scope9/1
  Sequence Analyzer8/1 -> Scope10/1
  Sequence Analyzer6/1 -> Scope8/1
  Sequence Analyzer9/1 -> Scope11/1
  Sequence Analyzer2/2 -> Terminator/1
  Sequence Analyzer7/2 -> Terminator7/1
  Sequence Analyzer6/2 -> Terminator8/1
  Sequence Analyzer8/2 -> Terminator6/1
  Sequence Analyzer/2 -> Terminator2/1
  Sequence Analyzer1/2 -> Terminator1/1
  Sequence Analyzer5/2 -> Terminator3/1
  Sequence Analyzer4/2 -> Terminator4/1
  Sequence Analyzer3/2 -> Terminator5/1
  Sequence Analyzer/1 -> Scope2/1
  Sequence Analyzer2/1 -> Scope4/1
  Sequence Analyzer9/2 -> Terminator9/1
  Sequence Analyzer1/1 -> Scope3/1
  abc/1 -> Sequence Analyzer3/1, Sequence Analyzer/1, Sequence Analyzer1/1, Sequence Analyzer2/1, Sequence Analyzer4/1, Sequence Analyzer5/1, Sequence Analyzer6/1, Sequence Analyzer7/1, Sequence Analyzer8/1, Sequence Analyzer9/1
  Sequence Analyzer5/1 -> Scope7/1
  Sequence Analyzer3/1 -> Scope5/1
  Sequence Analyzer4/1 -> Scope6/1

== system SPGF_FSK_0000_R2019b/TP15/Nonlinear Load ==
  Cap : powerlib/Elements/Series RLC Branch  LConnTagsString=__new0  RConnTagsString=__new0  BranchType=C  Resistance=34  Inductance=1.04  SetiL0=off  InitialCurrent=0  Capacitance=4e-06  Setx0=off  InitialVoltage=0  Measurements=None
  Cap1 : powerlib/Elements/Series RLC Branch  LConnTagsString=__new0  RConnTagsString=__new0  BranchType=C  Resistance=34  Inductance=1.04  SetiL0=off  InitialCurrent=0  Capacitance=4e-06  Setx0=off  InitialVoltage=0  Measurements=None
  Cap2 : powerlib/Elements/Series RLC Branch  LConnTagsString=__new0  RConnTagsString=__new0  BranchType=C  Resistance=34  Inductance=1.04  SetiL0=off  InitialCurrent=0  Capacitance=4e-06  Setx0=off  InitialVoltage=0  Measurements=None
  Ground : powerlib/Elements/Ground  LConnTagsString=a
  RL : powerlib/Elements/Series RLC Branch  LConnTagsString=__new0  RConnTagsString=__new0  BranchType=RL  Resistance=58  Inductance=1.04  SetiL0=off  InitialCurrent=0  Capacitance=1e-6  Setx0=off  InitialVoltage=0  Measurements=None
  RL1 : powerlib/Elements/Series RLC Branch  LConnTagsString=__new0  RConnTagsString=__new0  BranchType=RL  Resistance=40  Inductance=1.04  SetiL0=off  InitialCurrent=0  Capacitance=1e-6  Setx0=off  InitialVoltage=0  Measurements=None
  RL2 : powerlib/Elements/Series RLC Branch  LConnTagsString=__new0  RConnTagsString=__new0  BranchType=RL  Resistance=40  Inductance=1.04  SetiL0=off  InitialCurrent=0  Capacitance=1e-6  Setx0=off  InitialVoltage=0  Measurements=None
  Universal Bridge : powerlib/Power Electronics/Universal Bridge  Arms=2  SnubberResistance=1e5  SnubberCapacitance=inf  Device=Diodes  Ron=1e-3  Lon=0  ForwardVoltages="[  0  0  ]"  ForwardVoltage=-160  GTOparameters=[ 10e-6 , 20e-6 ]  IGBTparameters=[ 1e-6 , 2e-6 ]  Measurements=None  Measurements_2=None  converterType=Rectifier
  Universal Bridge1 : powerlib/Power Electronics/Universal Bridge  Arms=2  SnubberResistance=1e5  SnubberCapacitance=inf  Device=Diodes  Ron=1e-3  Lon=0  ForwardVoltages="[  0  0  ]"  ForwardVoltage=-160  GTOparameters=[ 10e-6 , 20e-6 ]  IGBTparameters=[ 1e-6 , 2e-6 ]  Measurements=None  Measurements_2=None  converterType=Rectifier
  Universal Bridge2 : powerlib/Power Electronics/Universal Bridge  Arms=2  SnubberResistance=1e5  SnubberCapacitance=inf  Device=Diodes  Ron=1e-3  Lon=0  ForwardVoltages="[  0  0  ]"  ForwardVoltage=-160  GTOparameters=[ 10e-6 , 20e-6 ]  IGBTparameters=[ 1e-6 , 2e-6 ]  Measurements=None  Measurements_2=None  converterType=Rectifier
  A : PMIOPort  Side=Left
  B : PMIOPort  Port=2  Side=Left
  C : PMIOPort  Port=3  Side=Left
  connections:
  Cap/LConn1 -- Universal Bridge/RConn1 -- RL/LConn1
  Cap/RConn1 -- RL/RConn1 -- Universal Bridge/RConn2
  Cap1/LConn1 -- Universal Bridge1/RConn1 -- RL1/LConn1
  Universal Bridge1/RConn2 -- RL1/RConn1 -- Cap1/RConn1
  Cap2/LConn1 -- Universal Bridge2/RConn1 -- RL2/LConn1
  Cap2/RConn1 -- Universal Bridge2/RConn2 -- RL2/RConn1
  Universal Bridge/LConn1 -- A/RConn1
  Universal Bridge1/LConn1 -- B/RConn1
  Universal Bridge2/LConn1 -- C/RConn1
  Ground/LConn1 -- Universal Bridge/LConn2 -- Universal Bridge1/LConn2 -- Universal Bridge2/LConn2

== system SPGF_FSK_0000_R2019b/TP15/Nonlinear Load 3ph ==
  Cap : powerlib/Elements/Series RLC Branch  LConnTagsString=__new0  RConnTagsString=__new0  BranchType=C  Resistance=34  Inductance=1.04  SetiL0=off  InitialCurrent=0  Capacitance=4e-06  Setx0=off  InitialVoltage=0  Measurements=None
  RL : powerlib/Elements/Series RLC Branch  LConnTagsString=__new0  RConnTagsString=__new0  BranchType=RL  Resistance=58  Inductance=1.04  SetiL0=off  InitialCurrent=0  Capacitance=1e-6  Setx0=off  InitialVoltage=0  Measurements=None
  Universal Bridge : powerlib/Power Electronics/Universal Bridge  Arms=3  SnubberResistance=1e5  SnubberCapacitance=inf  Device=Diodes  Ron=1e-3  Lon=0  ForwardVoltages="[  0  0  ]"  ForwardVoltage=-160  GTOparameters=[ 10e-6 , 20e-6 ]  IGBTparameters=[ 1e-6 , 2e-6 ]  Measurements=None  Measurements_2=None  converterType=Rectifier
  A : PMIOPort  Side=Left
  B : PMIOPort  Port=2  Side=Left
  C : PMIOPort  Port=3  Side=Left
  connections:
  Universal Bridge/RConn1 -- RL/LConn1 -- Cap/LConn1
  Cap/RConn1 -- Universal Bridge/RConn2 -- RL/RConn1
  Universal Bridge/LConn2 -- B/RConn1
  C/RConn1 -- Universal Bridge/LConn3
  A/RConn1 -- Universal Bridge/LConn1

== system SPGF_FSK_0000_R2019b/TP15/Q ==
  breaker : Subsystem  Commented=on  mask{SwitchA=off, SwitchB=off, SwitchC=off, InitialStatus=[1 1 1], BreakerResistance=0.0001, SnubberResistance=1e6, SnubberCapacitance=inf, TransitionTimes=[0.5 0.7], ShiftTimes=[0 0 0]}
      mask prompts: SwitchA "Switching of phase A"; SwitchB "Switching of phase B"; SwitchC "Switching of phase C"; InitialStatus "Initial status of phase breaker [A, B, C]"; BreakerResistance "Breaker resistance Ron (ohms) :"; SnubberResistance "Snubbers resistance Rp (ohms) :"; SnubberCapacitance "Snubbers capacitance Cp (F) :"; TransitionTimes "Transition times (s) :"; ShiftTimes "Time differences for switch [tA, tB, tC] (s) :"
      mask init: same as SPGF_FSK_0000_R2019b/Feed/Q/breaker
      mask Display:
      | % port_label('input',1,'Iabc');
      | 
      | port_label('lconn',1,'A');
      | port_label('lconn',2,'B');
      | port_label('lconn',3,'C');
      | 
      | port_label('rconn',1,'a');
      | port_label('rconn',2,'b');
      | port_label('rconn',3,'c');
      | 
      | disp('   Q    ');
  meas : Subsystem
  shunt : Subsystem
  A : PMIOPort  Side=Right
  B : PMIOPort  Port=2  Side=Right
  C : PMIOPort  Port=3  Side=Right
  a : PMIOPort  Port=4  Side=Left
  b : PMIOPort  Port=5  Side=Left
  c : PMIOPort  Port=6  Side=Left
  connections:
  shunt/LConn3 -- C/RConn1 -- breaker/LConn3
  shunt/LConn2 -- B/RConn1 -- breaker/LConn2
  A/RConn1 -- shunt/LConn1 -- breaker/LConn1
  meas/RConn1 -- a/RConn1
  meas/RConn2 -- b/RConn1
  meas/RConn3 -- c/RConn1
  meas/LConn3 -- breaker/RConn3 -- shunt/RConn3
  meas/LConn2 -- breaker/RConn2 -- shunt/RConn2
  meas/LConn1 -- breaker/RConn1 -- shunt/RConn1

== system SPGF_FSK_0000_R2019b/TP21/Nonlinear Load ==
  Cap : powerlib/Elements/Series RLC Branch  LConnTagsString=__new0  RConnTagsString=__new0  BranchType=C  Resistance=34  Inductance=1.04  SetiL0=off  InitialCurrent=0  Capacitance=4e-06  Setx0=off  InitialVoltage=0  Measurements=None
  Cap1 : powerlib/Elements/Series RLC Branch  LConnTagsString=__new0  RConnTagsString=__new0  BranchType=C  Resistance=34  Inductance=1.04  SetiL0=off  InitialCurrent=0  Capacitance=4e-06  Setx0=off  InitialVoltage=0  Measurements=None
  Cap2 : powerlib/Elements/Series RLC Branch  LConnTagsString=__new0  RConnTagsString=__new0  BranchType=C  Resistance=34  Inductance=1.04  SetiL0=off  InitialCurrent=0  Capacitance=4e-06  Setx0=off  InitialVoltage=0  Measurements=None
  Ground : powerlib/Elements/Ground  LConnTagsString=a
  RL : powerlib/Elements/Series RLC Branch  LConnTagsString=__new0  RConnTagsString=__new0  BranchType=RL  Resistance=58  Inductance=1.04  SetiL0=off  InitialCurrent=0  Capacitance=1e-6  Setx0=off  InitialVoltage=0  Measurements=None
  RL1 : powerlib/Elements/Series RLC Branch  LConnTagsString=__new0  RConnTagsString=__new0  BranchType=RL  Resistance=40  Inductance=1.04  SetiL0=off  InitialCurrent=0  Capacitance=1e-6  Setx0=off  InitialVoltage=0  Measurements=None
  RL2 : powerlib/Elements/Series RLC Branch  LConnTagsString=__new0  RConnTagsString=__new0  BranchType=RL  Resistance=40  Inductance=1.04  SetiL0=off  InitialCurrent=0  Capacitance=1e-6  Setx0=off  InitialVoltage=0  Measurements=None
  Universal Bridge : powerlib/Power Electronics/Universal Bridge  Arms=2  SnubberResistance=1e5  SnubberCapacitance=inf  Device=Diodes  Ron=1e-3  Lon=0  ForwardVoltages="[  0  0  ]"  ForwardVoltage=-160  GTOparameters=[ 10e-6 , 20e-6 ]  IGBTparameters=[ 1e-6 , 2e-6 ]  Measurements=None  Measurements_2=None  converterType=Rectifier
  Universal Bridge1 : powerlib/Power Electronics/Universal Bridge  Arms=2  SnubberResistance=1e5  SnubberCapacitance=inf  Device=Diodes  Ron=1e-3  Lon=0  ForwardVoltages="[  0  0  ]"  ForwardVoltage=-160  GTOparameters=[ 10e-6 , 20e-6 ]  IGBTparameters=[ 1e-6 , 2e-6 ]  Measurements=None  Measurements_2=None  converterType=Rectifier
  Universal Bridge2 : powerlib/Power Electronics/Universal Bridge  Arms=2  SnubberResistance=1e5  SnubberCapacitance=inf  Device=Diodes  Ron=1e-3  Lon=0  ForwardVoltages="[  0  0  ]"  ForwardVoltage=-160  GTOparameters=[ 10e-6 , 20e-6 ]  IGBTparameters=[ 1e-6 , 2e-6 ]  Measurements=None  Measurements_2=None  converterType=Rectifier
  A : PMIOPort  Side=Left
  B : PMIOPort  Port=2  Side=Left
  C : PMIOPort  Port=3  Side=Left
  connections:
  Cap/LConn1 -- Universal Bridge/RConn1 -- RL/LConn1
  Cap/RConn1 -- RL/RConn1 -- Universal Bridge/RConn2
  Cap1/LConn1 -- Universal Bridge1/RConn1 -- RL1/LConn1
  Universal Bridge1/RConn2 -- RL1/RConn1 -- Cap1/RConn1
  Cap2/LConn1 -- Universal Bridge2/RConn1 -- RL2/LConn1
  Cap2/RConn1 -- Universal Bridge2/RConn2 -- RL2/RConn1
  Universal Bridge/LConn1 -- A/RConn1
  Universal Bridge1/LConn1 -- B/RConn1
  Universal Bridge2/LConn1 -- C/RConn1
  Ground/LConn1 -- Universal Bridge/LConn2 -- Universal Bridge1/LConn2 -- Universal Bridge2/LConn2

== system SPGF_FSK_0000_R2019b/TP21/Nonlinear Load 3ph ==
  Cap : powerlib/Elements/Series RLC Branch  LConnTagsString=__new0  RConnTagsString=__new0  BranchType=C  Resistance=34  Inductance=1.04  SetiL0=off  InitialCurrent=0  Capacitance=4e-06  Setx0=off  InitialVoltage=0  Measurements=None
  RL : powerlib/Elements/Series RLC Branch  LConnTagsString=__new0  RConnTagsString=__new0  BranchType=RL  Resistance=58  Inductance=1.04  SetiL0=off  InitialCurrent=0  Capacitance=1e-6  Setx0=off  InitialVoltage=0  Measurements=None
  Universal Bridge : powerlib/Power Electronics/Universal Bridge  Arms=3  SnubberResistance=1e5  SnubberCapacitance=inf  Device=Diodes  Ron=1e-3  Lon=0  ForwardVoltages="[  0  0  ]"  ForwardVoltage=-160  GTOparameters=[ 10e-6 , 20e-6 ]  IGBTparameters=[ 1e-6 , 2e-6 ]  Measurements=None  Measurements_2=None  converterType=Rectifier
  A : PMIOPort  Side=Left
  B : PMIOPort  Port=2  Side=Left
  C : PMIOPort  Port=3  Side=Left
  connections:
  Universal Bridge/RConn1 -- RL/LConn1 -- Cap/LConn1
  Cap/RConn1 -- Universal Bridge/RConn2 -- RL/RConn1
  Universal Bridge/LConn2 -- B/RConn1
  C/RConn1 -- Universal Bridge/LConn3
  A/RConn1 -- Universal Bridge/LConn1

== system SPGF_FSK_0000_R2019b/TP21/Q ==
  breaker : Subsystem  Commented=on  mask{SwitchA=off, SwitchB=off, SwitchC=off, InitialStatus=[1 1 1], BreakerResistance=0.0001, SnubberResistance=1e6, SnubberCapacitance=inf, TransitionTimes=[0.5 0.7], ShiftTimes=[0 0 0]}
      mask prompts: SwitchA "Switching of phase A"; SwitchB "Switching of phase B"; SwitchC "Switching of phase C"; InitialStatus "Initial status of phase breaker [A, B, C]"; BreakerResistance "Breaker resistance Ron (ohms) :"; SnubberResistance "Snubbers resistance Rp (ohms) :"; SnubberCapacitance "Snubbers capacitance Cp (F) :"; TransitionTimes "Transition times (s) :"; ShiftTimes "Time differences for switch [tA, tB, tC] (s) :"
      mask init: same as SPGF_FSK_0000_R2019b/Feed/Q/breaker
      mask Display:
      | % port_label('input',1,'Iabc');
      | 
      | port_label('lconn',1,'A');
      | port_label('lconn',2,'B');
      | port_label('lconn',3,'C');
      | 
      | port_label('rconn',1,'a');
      | port_label('rconn',2,'b');
      | port_label('rconn',3,'c');
      | 
      | disp('   Q    ');
  meas : Subsystem
  shunt : Subsystem
  A : PMIOPort  Side=Right
  B : PMIOPort  Port=2  Side=Right
  C : PMIOPort  Port=3  Side=Right
  a : PMIOPort  Port=4  Side=Left
  b : PMIOPort  Port=5  Side=Left
  c : PMIOPort  Port=6  Side=Left
  connections:
  shunt/LConn3 -- C/RConn1 -- breaker/LConn3
  shunt/LConn2 -- B/RConn1 -- breaker/LConn2
  A/RConn1 -- shunt/LConn1 -- breaker/LConn1
  meas/RConn1 -- a/RConn1
  meas/RConn2 -- b/RConn1
  meas/RConn3 -- c/RConn1
  meas/LConn3 -- breaker/RConn3 -- shunt/RConn3
  meas/LConn2 -- breaker/RConn2 -- shunt/RConn2
  meas/LConn1 -- breaker/RConn1 -- shunt/RConn1
